simulink model "ReferenceTrajectoryExample"  (R2014b)
settings: Solver=ode45  StartTime=0.0  StopTime=10.0  RelTol=1e-3
settings Model: Creator=tchoopojcharoen  LastModifiedBy=tchoopojcharoen

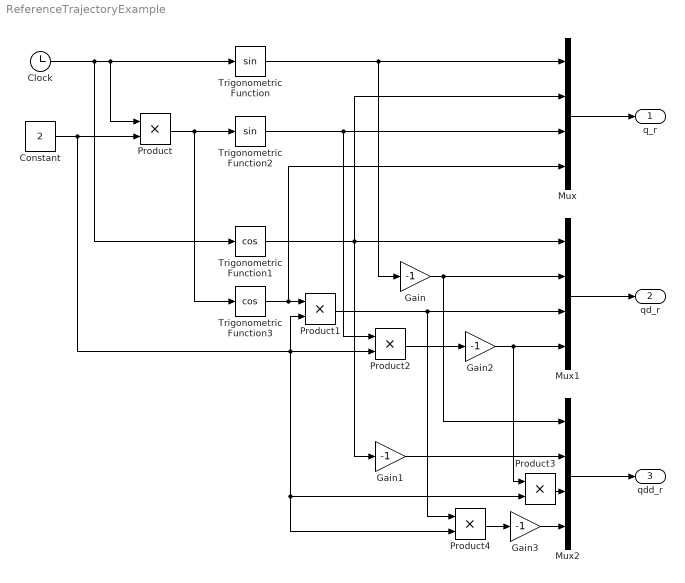
== system ReferenceTrajectoryExample ==
  Clock : Clock
  Constant : Constant  Value=2
  Gain{,1..3} (4 alike) : Gain  Gain=-1
  Mux : Mux
  Mux1 : Mux
  Mux2 : Mux
  Product{,1..4} (5 alike) : Product
  Trigonometric Function : Trigonometry
  Trigonometric Function1 : Trigonometry  Operator=cos
  Trigonometric Function2 : Trigonometry
  Trigonometric Function3 : Trigonometry  Operator=cos
  q_r : Outport
  qd_r : Outport  Port=2
  qdd_r : Outport  Port=3
  wires:
  Clock/1 -> Trigonometric Function/1, Product/1, Trigonometric Function1/1
  Trigonometric Function/1 -> Gain/1, Mux/1
  Trigonometric Function1/1 -> Gain1/1, Mux1/1, Mux/2
  Gain/1 -> Mux2/1, Mux1/2
  Gain1/1 -> Mux2/2
  Constant/1 -> Product4/2, Product3/2, Product2/2, Product1/2, Product/2
  Product/1 -> Trigonometric Function2/1, Trigonometric Function3/1
  Trigonometric Function2/1 -> Product2/1, Mux/3
  Product1/1 -> Mux1/3, Product4/1
  Trigonometric Function3/1 -> Mux/4, Product1/1
  Gain2/1 -> Product3/1, Mux1/4
  Product2/1 -> Gain2/1
  Product3/1 -> Mux2/3
  Product4/1 -> Gain3/1
  Gain3/1 -> Mux2/4
  Mux/1 -> q_r/1
  Mux1/1 -> qd_r/1
  Mux2/1 -> qdd_r/1
